simulink model "TrajectoryPlanningModel"  (R2020b)
settings: Solver=VariableStepAuto  StartTime=0.0  StopTime=10.0  RelTol=1e-3
values from neighbouring files (symbols this model uses):
  L0 = z(7)    [Forward_kinematics.m]    (also in GeometricCalculation_simulink.m = Geoparams(4); PRBDM_3R_parameters.m = 0.03; PRBDM_3R_parameters.mat = 0.03; TrajectoryPlanning_simulink.m = X(8))
  L1 = z(8)    [Forward_kinematics.m]    (also in GeometricCalculation_simulink.m = Geoparams(5); Jacobi.m = x(4); PRBDM_3R_CTC.m = x(19); PRBDM_3R_Dynamic_Matrices_NewtonEular.m = robot_params(4))
  L2 = z(9)    [Forward_kinematics.m]    (also in GeometricCalculation_simulink.m = Geoparams(6); Jacobi.m = x(5); PRBDM_3R_CTC.m = x(20); PRBDM_3R_Dynamic_Matrices_NewtonEular.m = robot_params(5))
  phi = pi/3    (= 1.0471975512)    [PRBDM_3R_test001.m]
  xd = 0.0536    [PRBDM_3R_test001.m]    (also in PRBDM_CTC_task.m = z(13); RRR_CTC_task.m = z(13))
  yd = 0.0135    [PRBDM_3R_test001.m]    (also in PRBDM_CTC_task.m = z(14); RRR_CTC_task.m = z(14))
settings Model: Creator=Master  LastModifiedBy=Master
settings DebuggingCC: UnderSpecifiedDimensionMsg=error

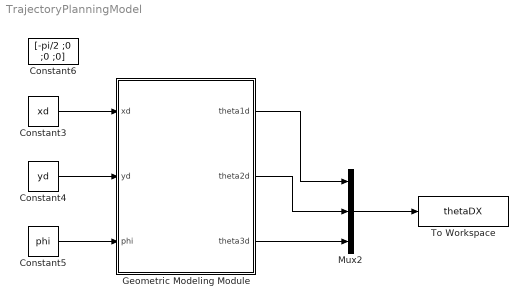
== system TrajectoryPlanningModel ==
  Constant3 : Constant  Value=xd
  Constant4 : Constant  Value=yd
  Constant5 : Constant  Value=phi
  Constant6 : Constant  Value=[-pi/2 ;0 ;0 ;0]
  Geometric Modeling Module : Subsystem
  Mux2 : Mux  Inputs=3
  To Workspace : ToWorkspace  VariableName=thetaDX  SaveFormat=Timeseries  SampleTime=-1
  wires:
  Constant4/1 -> Geometric Modeling Module/2(yd)
  Constant5/1 -> Geometric Modeling Module/3(phi)
  Constant3/1 -> Geometric Modeling Module/1(xd)
  Geometric Modeling Module/1(theta1d) -> Mux2/1
  Geometric Modeling Module/2(theta2d) -> Mux2/2
  Geometric Modeling Module/3(theta3d) -> Mux2/3
  Mux2/1 -> To Workspace/1

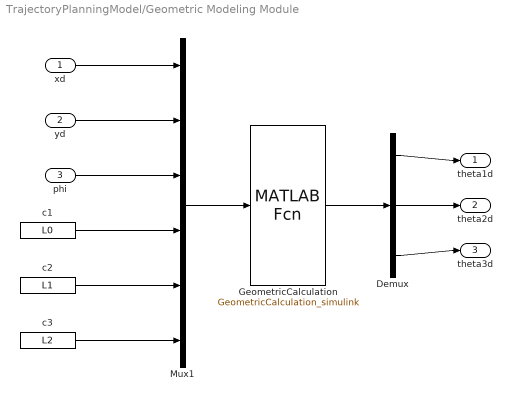
== system TrajectoryPlanningModel/Geometric Modeling Module ==
  xd : Inport
  yd : Inport  Port=2
  phi : Inport  Port=3
  Demux : Demux  Outputs=3
  GeometricCalculation : MATLABFcn  MATLABFcn=GeometricCalculation_simulink
  Mux1 : Mux  Inputs=6
  c1 : Constant  Value=L0
  c2 : Constant  Value=L1
  c3 : Constant  Value=L2
  theta1d : Outport
  theta2d : Outport  Port=2
  theta3d : Outport  Port=3
  wires:
  Mux1/1 -> GeometricCalculation/1
  yd/1 -> Mux1/2
  xd/1 -> Mux1/1
  phi/1 -> Mux1/3
  c1/1 -> Mux1/4
  c3/1 -> Mux1/6
  c2/1 -> Mux1/5
  GeometricCalculation/1 -> Demux/1
  Demux/2 -> theta2d/1
  Demux/1 -> theta1d/1
  Demux/3 -> theta3d/1
